simulink library "quanser_aero"  (R2019b)
settings: Solver=ode1  StartTime=0.0  StopTime=inf  FixedStep=0.002  RelTol=1e-3  EnableMultiTasking=on
undefined symbols (not defined in the file): HIL
libraries: quarc_library x3
settings Model: ExtModeTrigDuration=5000  Creator=MLevis  LastModifiedBy=johannes
settings SolverCC: PositivePriorityOrder=on
settings DataIOCC: LimitDataPoints=on  SaveFormat=Array  ReturnWorkspaceOutputs=off
settings OptimizationCC: LifeSpan=inf
settings DebuggingCC: SolverPrmCheckMsg=warning  SFUnexpectedBacktrackingDiag=warning  SFNoUnconditionalDefaultTransitionDiag=warning  SFExecutionAtInitializationDiag=none  ArithmeticOperatorsInVariantConditions=warning
settings HardwareCC: ProdBitPerPointer=32  ProdBitPerSizeT=32  ProdBitPerPtrDiffT=32  ProdLargestAtomicFloat=None  ProdIntDivRoundTo=Undefined  ProdEndianess=Unspecified  ProdWordSize=32  ProdHWDeviceType=32-bit Generic
settings ModelReferenceCC: PropagateSignalLabelsOutOfModel=off
settings SFSimCC: SimUseLocalCustomCode=off  CustomCodeUndefinedFunction=UseInterfaceOnly
settings RTWCC: Description=QUARC Win64 Target  SystemTargetFile=quarc_win64.tlc  TemplateMakefile=quarc_default_tmf  RTWUseLocalCustomCode=off
settings CodeAppCC: StateflowObjectComments=on
settings STFCustomTargetCC: TargetPreCompLibLocation=C:\PROGRA~3\QUARC\lib\2014a\win64\release  ConcurrentExecutionCompliant=on  GeneratePreprocessorConditionals=Disable all  GRTInterface=on  SystemTargetFile=quarc_win64.tlc
settings GRTTargetCC: TargetPreCompLibLocation=C:\PROGRA~3\QUARC\lib\2014a\win64\release  TargetLangStandard=C89/C90 (ANSI)  ParMdlRefBuildCompliant=off  CompOptLevelCompliant=off  GeneratePreprocessorConditionals=Disable all  CombineOutputUpdateFcns=off  MatFileLogging=off  CPPClassGenCompliant=off  GRTInterface=on  UseToolchainInfoCompliant=off  ExtMode=on  ExtModeMexFile=quarc_comm
settings ConfigComp: CovMetricSettings=dw  CovHtmlReporting=on  CovSaveCumulativeToWorkspaceVar=on  CovSaveSingleToWorkspaceVar=on  CovExternalEMLEnable=off  CovSFcnEnable=off

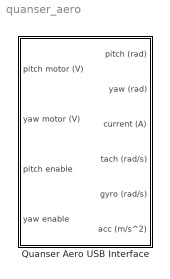
== system quanser_aero ==
  Quanser Aero USB Interface : Subsystem

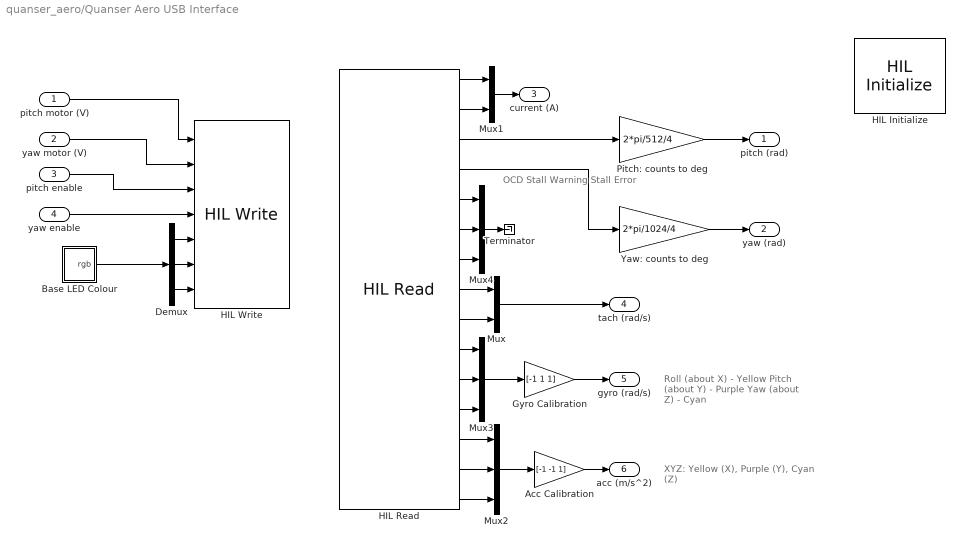
== system quanser_aero/Quanser Aero USB Interface ==
  note: Roll (about X) - Yellow
      | Pitch (about Y) - Purple
      | Yaw (about Z) - Cyan
  note: XYZ:
      | Yellow (X), Purple (Y), Cyan (Z)
  note: OCD
      | Stall Warning
      | Stall Error
  pitch motor (V) : Inport
  yaw motor (V) : Inport  Port=2
  pitch enable : Inport  Port=3
  yaw enable : Inport  Port=4
  Acc Calibration : Gain  Gain=[-1 -1 1]
  Base LED Colour : Subsystem  mask(Color Constant){color=[0 1 0]}
      mask help: Outputs a constant RGB color value.
      mask init:
      | rgb = get_param(gcbh, 'color');
      | if numel(color) ~= 3
      |     rgb = [0 0 0];
      | end
      | set_param(gcbh, 'MaskDisplay', ['patch([-0.02 -0.02 1.02 1.02], [-0.02 1.02 1.02 -0.02], ', rgb, ');']);
      settings: OpenFcn=color_constant_properties('CurrentBlock', gcbh);
      mask Help: web(qc_get_block_help_path(gcb), '-helpbrowser');
      mask Display: patch([-0.02 -0.02 1.02 1.02], [-0.02 1.02 1.02 -0.02], [0 1 0]);
  Demux : Demux  Outputs=3
  Gyro Calibration : Gain  Gain=[-1 1 1]
  HIL Initialize : quarc_library/Data Acquisition/Generic/Configuration/HIL Initialize  Priority=-99  object_name=HIL-1  board_type=quanser_aero_usb  board_number=0  board_options=""  exclusive=off  active=off  hardware_clocks=[0]  clock_modes=[]  initial_clock_frequencies=[]  set_clock_params_at_start=off  set_clock_params_at_switch_in=off  set_clock_frequencies_at_start=off  set_clock_frequencies_at_switch_in=off  analog_input_channels=[0:1]  analog_input_maximums=3  analog_input_minimums=-3  set_analog_input_params_at_start=off  set_analog_input_params_at_switch_in=off  analog_output_channels=[0:1]  analog_output_maximums=24  analog_output_minimums=-24  initial_analog_outputs=[0]  final_analog_outputs=[0]  watchdog_analog_outputs=[0]  set_analog_output_params_at_start=off  set_analog_output_params_at_switch_in=off  set_analog_outputs_at_start=on  set_analog_outputs_at_switch_in=off  set_analog_outputs_at_terminate=on  set_analog_outputs_at_switch_out=off  set_analog_outputs_on_watchdog=on  digital_input_channels=[]  digital_output_channels=[0:1]  digital_output_configuration=[]  initial_digital_outputs=[1]  final_digital_outputs=[0]  watchdog_digital_outputs=[0]  set_digital_output_params_at_start=off  set_digital_output_params_at_switch_in=off  set_digital_outputs_at_start=on  set_digital_outputs_at_switch_in=off  set_digital_outputs_at_terminate=on  set_digital_outputs_at_switch_out=off  set_digital_outputs_on_watchdog=on  encoder_channels=[0:3]  quadrature=[4]  encoder_filter_frequency=[]  initial_encoder_counts=[0]  set_encoder_params_at_start=off  set_encoder_params_at_switch_in=off  set_encoder_counts_at_start=on  set_encoder_counts_at_switch_in=off  pwm_channels=[]  pwm_modes=[]  pwm_frequency=[]  pwm_configuration=[]  pwm_alignment=[]  pwm_polarity=[]  pwm_leading_deadband=[]  pwm_trailing_deadband=[]  initial_pwm_outputs=[]  final_pwm_outputs=[]  watchdog_pwm_outputs=[]  set_pwm_params_at_start=off  set_pwm_params_at_switch_in=off  set_pwm_outputs_at_start=off  set_pwm_outputs_at_switch_in=off  set_pwm_outputs_at_terminate=off  set_pwm_outputs_at_switch_out=off  set_pwm_outputs_on_watchdog=off  other_output_channels=[11000:11002]  initial_other_outputs=[0 1 0]  final_other_outputs=[1 0 0]  watchdog_other_outputs=[0 0 1]  set_other_outputs_at_start=on  set_other_outputs_at_switch_in=off  set_other_outputs_at_terminate=on  set_other_outputs_at_switch_out=off  set_other_outputs_on_watchdog=on
  HIL Read : quarc_library/Data Acquisition/Generic/Immediate I//O/HIL Read  object_name=HIL-1  analog_channels=[0:1]  encoder_channels=[2:3]  digital_channels=[0:2]  other_channels=[14000:14001 3000:3002 4000:4002]  sample_time=qc_get_step_size  active=on  vector_output=off  data_type_mode=Inherit via back propagation  encoder_data_type=double  digital_data_type=boolean
  HIL Write : quarc_library/Data Acquisition/Generic/Immediate I//O/HIL Write  object_name=HIL-1  analog_channels=[0:1]  pwm_channels=[]  digital_channels=[0:1]  other_channels=[11000:11002]  sample_time=-1  active=off  vector_input=off
  Mux : Mux  Inputs=2
  Mux1 : Mux  Inputs=2
  Mux2 : Mux  Inputs=3
  Mux3 : Mux  Inputs=3
  Mux4 : Mux  Inputs=3
  Pitch: counts to deg : Gain  Gain=2*pi/512/4
  Terminator : Terminator
  Yaw: counts to deg : Gain  Gain=2*pi/1024/4
  pitch (rad) : Outport
  yaw (rad) : Outport  Port=2
  current (A) : Outport  Port=3
  tach (rad/s) : Outport  Port=4
  gyro (rad/s) : Outport  Port=5
  acc (m/s^2) : Outport  Port=6
  wires:
  Mux2/1 -> Acc Calibration/1
  pitch enable/1 -> HIL Write/3
  yaw enable/1 -> HIL Write/4
  Base LED Colour/1(rgb) -> Demux/1
  Demux/1 -> HIL Write/5
  Demux/2 -> HIL Write/6
  Demux/3 -> HIL Write/7
  HIL Read/1 -> Mux1/1
  HIL Read/2 -> Mux1/2
  Yaw: counts to deg/1 -> yaw (rad)/1
  Pitch: counts to deg/1 -> pitch (rad)/1
  pitch motor (V)/1 -> HIL Write/1
  Mux1/1 -> current (A)/1
  HIL Read/3 -> Pitch: counts to deg/1
  HIL Read/4 -> Yaw: counts to deg/1
  Mux3/1 -> Gyro Calibration/1
  Gyro Calibration/1 -> gyro (rad/s)/1
  yaw motor (V)/1 -> HIL Write/2
  Mux/1 -> tach (rad/s)/1
  HIL Read/15 -> Mux2/3
  HIL Read/14 -> Mux2/2
  HIL Read/13 -> Mux2/1
  HIL Read/10 -> Mux3/1
  HIL Read/11 -> Mux3/2
  HIL Read/12 -> Mux3/3
  HIL Read/8 -> Mux/1
  HIL Read/9 -> Mux/2
  HIL Read/5 -> Mux4/1
  HIL Read/6 -> Mux4/2
  HIL Read/7 -> Mux4/3
  Mux4/1 -> Terminator/1
  Acc Calibration/1 -> acc (m/s^2)/1

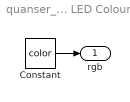
== system quanser_aero/Quanser Aero USB Interface/Base LED Colour ==
  Constant : Constant  Value=color
  rgb : Outport
  wires:
  Constant/1 -> rgb/1
